simulink model "ece456prob3"  (R2017a)
settings: Solver=VariableStepAuto  StartTime=0.0  StopTime=4.0  RelTol=1e-3
settings Model: Creator=b  LastModifiedBy=b

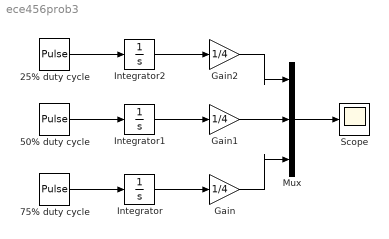
== system ece456prob3 ==
  25% duty cycle : DiscretePulseGenerator  PulseType=Time based  Amplitude=4  Period=4  PulseWidth=25
  50% duty cycle : DiscretePulseGenerator  PulseType=Time based  Amplitude=4  Period=4  PulseWidth=50
  75% duty cycle : DiscretePulseGenerator  PulseType=Time based  Amplitude=4  Period=4  PulseWidth=75
  Gain : Gain  Gain=1/4
  Gain1 : Gain  Gain=1/4
  Gain2 : Gain  Gain=1/4
  Integrator : Integrator
  Integrator1 : Integrator
  Integrator2 : Integrator
  Mux : Mux  Inputs=3
  Scope : Scope
  wires:
  75% duty cycle/1 -> Integrator/1
  Integrator/1 -> Gain/1
  Gain1/1 -> Mux/2
  50% duty cycle/1 -> Integrator1/1
  Integrator1/1 -> Gain1/1
  Gain2/1 -> Mux/1
  25% duty cycle/1 -> Integrator2/1
  Integrator2/1 -> Gain2/1
  Gain/1 -> Mux/3
  Mux/1 -> Scope/1
